simulink model "GT_TECS"  (R2024a)
settings: Solver=ode4  StartTime=0.0  StopTime=100  FixedStep=1/1600  RelTol=1e-3
undefined symbols (not defined in the file): Earth, euler0, H0, IMU_Freq, PTCH_Freq, U0, V0, WGS84, wind_x, wind_y, wind_z
libraries: Sensors x3, aerolibactuator x2, AP_PitchController x1, GT x1, aerolibtransform2 x1, aerolibnav x1, TECS x1
settings Model: Creator=igmso  LastModifiedBy=igmso
settings DataIOCC: ExternalInput=[t,u]  InitialState=getstatestruct(op_trim3)  SaveFormat=StructureWithTime

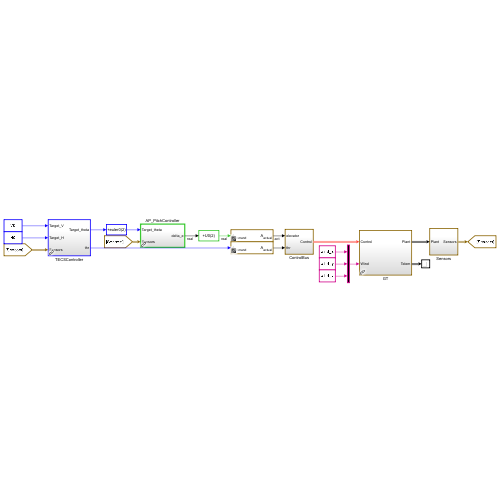
[thumbnail: Simulink's stored preview of the top-level diagram]
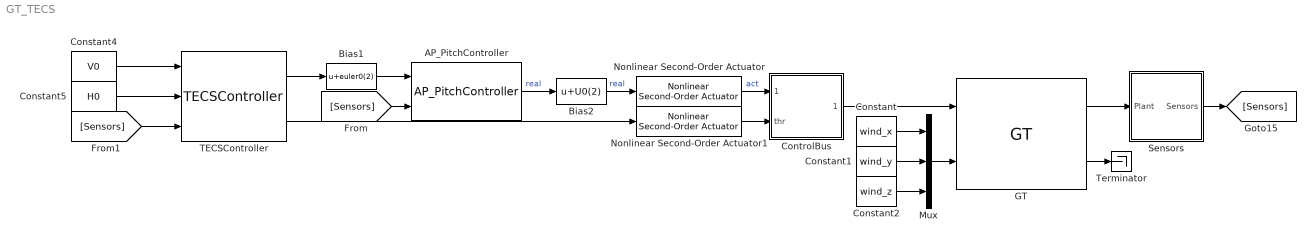
== system GT_TECS ==
  AP_PitchController : AP_PitchController/AP_PitchController  SystemSampleTime=1/PTCH_Freq  VariantActivationTime=update diagram  AllowFlexibleInterface=on  Latency=0  AutoFrameSizeCalculation=off
  Bias1 : Bias  Bias=euler0(2)  SaturateOnIntegerOverflow=off
  Bias2 : Bias  Bias=U0(2)  SaturateOnIntegerOverflow=off
  Constant : Constant  Value=wind_x
  Constant1 : Constant  Value=wind_y
  Constant2 : Constant  Value=wind_z
  Constant4 : Constant  Value=V0  SampleTime=-1
  Constant5 : Constant  Value=H0  SampleTime=-1
  ControlBus : Subsystem
  GT : GT/GT  SystemSampleTime=-1  VariantActivationTime=update diagram  AllowFlexibleInterface=on  Latency=0  AutoFrameSizeCalculation=off
  Mux : Mux  Inputs=3
  Nonlinear Second-Order Actuator : aerolibactuator/Nonlinear Second-Order Actuator  wn_fin=2  z_fin=0.7  fin_max=30  fin_min=-30  fin_maxrate=400  fin_act_0=0  fin_act_vel=0
  Nonlinear Second-Order Actuator1 : aerolibactuator/Nonlinear Second-Order Actuator  wn_fin=60  z_fin=0.7  fin_max=1  fin_min=0  fin_maxrate=50  fin_act_0=0  fin_act_vel=0
  Sensors : Subsystem
  TECSController : TECS/TECSController  SystemSampleTime=-1  VariantActivationTime=update diagram  AllowFlexibleInterface=on  Latency=0  AutoFrameSizeCalculation=off
  Terminator : Terminator
  wires:
  Mux/1 -> GT/2
  Constant/1 -> Mux/1
  Constant1/1 -> Mux/2
  Constant2/1 -> Mux/3
  GT/2 -> Terminator/1
  GT/1 -> Sensors/1(Plant)
  Sensors/1(Sensors) -> [Sensors]
  ControlBus/1(Control) -> GT/1
  Nonlinear Second-Order Actuator/1 -> ControlBus/1(elevator)  "act"
  [Sensors] -> AP_PitchController/2
  Nonlinear Second-Order Actuator1/1 -> ControlBus/2(thr)
  TECSController/1 -> Bias1/1
  [Sensors] -> TECSController/3
  TECSController/2 -> Nonlinear Second-Order Actuator1/1
  Bias1/1 -> AP_PitchController/1
  AP_PitchController/1 -> Bias2/1  "real"
  Bias2/1 -> Nonlinear Second-Order Actuator/1  "real"
  Constant4/1 -> TECSController/1
  Constant5/1 -> TECSController/2

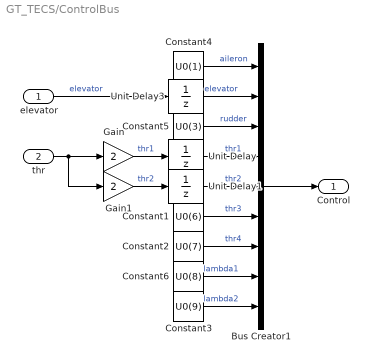
== system GT_TECS/ControlBus ==
  elevator : Inport
  thr : Inport  Port=2
  Bus Creator1 : BusCreator  Inputs=9
  Constant1 : Constant  Value=U0(6)  SampleTime=-1
  Constant2 : Constant  Value=U0(7)  SampleTime=-1
  Constant3 : Constant  Value=U0(9)  SampleTime=-1
  Constant4 : Constant  Value=U0(1)  SampleTime=-1
  Constant5 : Constant  Value=U0(3)  SampleTime=-1
  Constant6 : Constant  Value=U0(8)  SampleTime=-1
  Gain : Gain  Gain=2
  Gain1 : Gain  Gain=2
  Unit Delay : UnitDelay  InitialCondition=U0(4)  SampleTime=-1  HasFrameUpgradeWarning=on
  Unit Delay1 : UnitDelay  InitialCondition=U0(5)  SampleTime=-1  HasFrameUpgradeWarning=on
  Unit Delay3 : UnitDelay  SampleTime=-1  HasFrameUpgradeWarning=on
  Control : Outport
  wires:
  elevator/1 -> Unit Delay3/1  "elevator"
  Constant5/1 -> Bus Creator1/3  "rudder"
  Constant6/1 -> Bus Creator1/8  "lambda1"
  Constant3/1 -> Bus Creator1/9  "lambda2"
  Bus Creator1/1 -> Control/1
  Gain/1 -> Unit Delay/1  "thr1"
  Gain1/1 -> Unit Delay1/1  "thr2"
  Constant1/1 -> Bus Creator1/6  "thr3"
  Constant2/1 -> Bus Creator1/7  "thr4"
  Constant4/1 -> Bus Creator1/1  "aileron"
  thr/1 -> Gain1/1, Gain/1
  Unit Delay/1 -> Bus Creator1/4  "thr1"
  Unit Delay1/1 -> Bus Creator1/5  "thr2"
  Unit Delay3/1 -> Bus Creator1/2  "elevator"

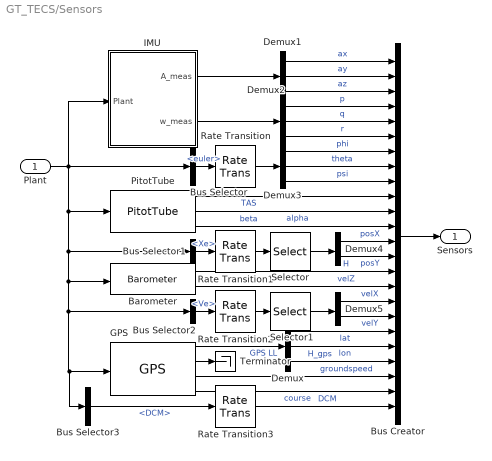
== system GT_TECS/Sensors ==
  Plant : Inport
  Barometer : Sensors/Barometer  SystemSampleTime=1/400  VariantActivationTime=update diagram  AllowFlexibleInterface=on  Latency=0  AutoFrameSizeCalculation=off
  Bus Selector : BusSelector  OutputSignals=euler
  Bus Selector1 : BusSelector  OutputSignals=Xe
  Bus Selector2 : BusSelector  OutputSignals=Ve
  Bus Selector3 : BusSelector  OutputSignals=DCM
  Bus Creator : BusCreator  Inputs=24
  Demux{,1..3} (4 alike) : Demux  Outputs=3
  Demux4 : Demux  Outputs=2
  Demux5 : Demux  Outputs=2
  GPS : Sensors/GPS  SystemSampleTime=1/10  VariantActivationTime=update diagram  AllowFlexibleInterface=on  Latency=0  AutoFrameSizeCalculation=off
  IMU : Subsystem  AncestorBlock=Sensors/IMU  TreatAsAtomicUnit=on
  PitotTube : Sensors/PitotTube  SystemSampleTime=1/400  VariantActivationTime=update diagram  AllowFlexibleInterface=on  Latency=0  AutoFrameSizeCalculation=off
  Rate Transition{,1..3} (4 alike) : RateTransition  OutPortSampleTime=1/IMU_Freq
  Selector : Selector  InputPortWidth=3  IndexOptions=Index vector (dialog)  Indices=[1 2]  OutputSizes=1
  Selector1 : Selector  InputPortWidth=3  IndexOptions=Index vector (dialog)  Indices=[1 2]  OutputSizes=1
  Terminator : Terminator
  Sensors : Outport
  wires:
  Barometer/1 -> Bus Creator/15  "H"
  GPS/2 -> Terminator/1
  GPS/3 -> Bus Creator/22  "groundspeed"
  GPS/4 -> Bus Creator/23  "course"
  Demux/1 -> Bus Creator/19  "lat"
  Demux/2 -> Bus Creator/20  "lon"
  Demux/3 -> Bus Creator/21  "H_gps"
  PitotTube/1 -> Bus Creator/10  "TAS"
  PitotTube/2 -> Bus Creator/11  "alpha"
  PitotTube/3 -> Bus Creator/12  "beta"
  Demux1/3 -> Bus Creator/3  "az"
  Demux1/2 -> Bus Creator/2  "ay"
  Demux1/1 -> Bus Creator/1  "ax"
  IMU/1(A_meas) -> Demux1/1
  IMU/2(w_meas) -> Demux2/1
  Demux2/1 -> Bus Creator/4  "p"
  Demux2/2 -> Bus Creator/5  "q"
  Demux2/3 -> Bus Creator/6  "r"
  Barometer/2 -> Bus Creator/16  "velZ"
  GPS/1 -> Demux/1  "GPS LL"
  Bus Selector/1 -> Rate Transition/1  "<euler>"
  Demux3/1 -> Bus Creator/7  "phi"
  Demux3/2 -> Bus Creator/8  "theta"
  Demux3/3 -> Bus Creator/9  "psi"
  Bus Selector1/1 -> Rate Transition1/1  "<Xe>"
  Selector/1 -> Demux4/1
  Demux4/1 -> Bus Creator/13  "posX"
  Demux4/2 -> Bus Creator/14  "posY"
  Bus Creator/1 -> Sensors/1
  Selector1/1 -> Demux5/1
  Bus Selector2/1 -> Rate Transition2/1  "<Ve>"
  Plant/1 -> IMU/1(Plant), Bus Selector2/1, Bus Selector3/1, GPS/1, Barometer/1, Bus Selector1/1, PitotTube/1, Bus Selector/1
  Demux5/1 -> Bus Creator/17  "velX"
  Demux5/2 -> Bus Creator/18  "velY"
  Rate Transition/1 -> Demux3/1
  Rate Transition1/1 -> Selector/1
  Rate Transition2/1 -> Selector1/1
  Bus Selector3/1 -> Rate Transition3/1  "<DCM>"
  Rate Transition3/1 -> Bus Creator/24  "DCM"

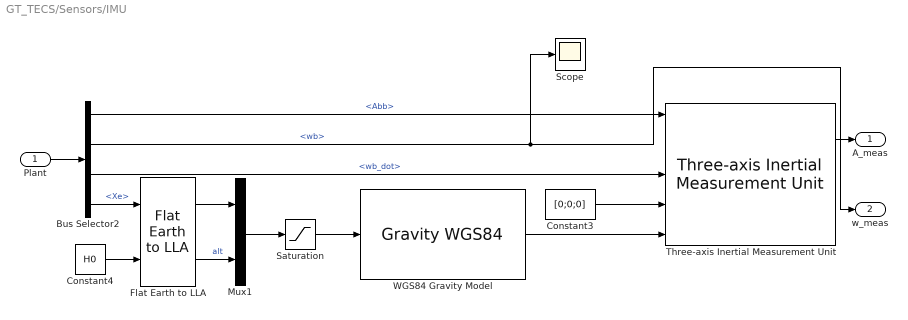
== system GT_TECS/Sensors/IMU ==
  Plant : Inport  SampleTime=1/IMU_Freq
  Bus Selector2 : BusSelector  OutputSignals=Abb,wb,wb_dot,Xe
  Constant3 : Constant  Value=[0;0;0]  SampleTime=1/IMU_Freq
  Constant4 : Constant  Value=H0  SampleTime=1/IMU_Freq
  Flat Earth to LLA : aerolibtransform2/Flat Earth to LLA  units=Metric (MKS)  ptype=Earth (WGS84)  F=1/298.257223563  R=6378137  refPosPort=off  LL0=SJK_airport  psi=SJK_direction
  Mux1 : Mux  Inputs=2
  Saturation : Saturate  UpperLimit=2033  LowerLimit=0
  Scope : Scope
  Three-axis Inertial Measurement Unit : aerolibnav/Three-axis Inertial Measurement Unit  units=Metric (MKS)  imu=[0 0 0]  i_Ts=1/800  dtype_a=off  w_a=190  z_a=0.707  a_sf_cc=[1 0 0; 0 1 0; 0 0 1]  a_bias=[0 0 0]  a_sat="[-inf  -inf  -inf  inf inf inf]"  dtype_g=off  w_g=190  z_g=0.707  g_sf_cc=[1 0 0; 0 1 0; 0 0 1]  g_bias=[0 0 0]  g_sens=[0 0 0]  g_sat="[-inf  -inf  -inf  inf inf inf]"  i_rand=off  i_seeds=[23093 23094 23095 23096 23097 23098]  i_pow=[0.00001 0.00001 0.00001 0.000001 0.000001 0.000001]
  "WGS84 Gravity Model  " : GravityWGS84
  A_meas : Outport  SampleTime=1/IMU_Freq
  w_meas : Outport  Port=2  SampleTime=1/IMU_Freq
  wires:
  Bus Selector2/2 -> Scope/1, w_meas/1  "<wb>"
  Constant3/1 -> Three-axis Inertial Measurement Unit/4
  Bus Selector2/3 -> Three-axis Inertial Measurement Unit/3  "<wb_dot>"
  Mux1/1 -> Saturation/1
  Plant/1 -> Bus Selector2/1
  Bus Selector2/4 -> Flat Earth to LLA/1  "<Xe>"
  "WGS84 Gravity Model  "/1 -> Three-axis Inertial Measurement Unit/5
  Bus Selector2/1 -> Three-axis Inertial Measurement Unit/1  "<Abb>"
  Flat Earth to LLA/2 -> Mux1/2  "alt"
  Constant4/1 -> Flat Earth to LLA/2
  Flat Earth to LLA/1 -> Mux1/1
  Three-axis Inertial Measurement Unit/1 -> A_meas/1
  Saturation/1 -> "WGS84 Gravity Model  "/1
